simulink model "Bringup"  (R2024b)
settings: Solver=FixedStepDiscrete  StartTime=0.0  StopTime=Inf  FixedStep=Ts0  RelTol=1e-3  EnableMultiTasking=on
undefined symbols (not defined in the file): Omega, Ts0, Ts0Single
libraries: svdschedulerlib x1
settings Model: DataDictionary=RectData.sldd  VariantConfigurationObject=Conf  ExtModeTrigDuration=8  Creator=sgade  LastModifiedBy=sgade
settings SolverCC: AutoInsertRateTranBlk=on
settings OptimizationCC: DefaultUnderspecifiedDataType=single  EnhancedBackFolding=on  PassReuseOutputArgsAs=Individual arguments  MaxStackSize=1024  OptimizeBlockOrder=speed  DifferentSizesBufferReuse=on  OptimizationCustomize=off  EfficientTunableParamExpr=on
settings DebuggingCC: ParameterTunabilityLossMsg=error
settings HardwareCC: ProdBitPerChar=16  ProdBitPerInt=16  ProdBitPerPointer=32  ProdBitPerSizeT=32  ProdBitPerPtrDiffT=32  ProdLargestAtomicInteger=Integer  ProdLargestAtomicFloat=None  ProdWordSize=16  ProdLongLongMode=on  ProdHWDeviceType=Texas Instruments->C2000
settings SFSimCC: MATLABDynamicMemAlloc=off
settings RTWCC: Description=Embedded Coder  SystemTargetFile=ert.tlc  HardwareBoard=TI F280013x  TemplateMakefile=ert_default_tmf  Toolchain=Texas Instruments Code Composer Studio (C2000)  CodeProfilingSaveOptions=MetricsOnly
settings CodeAppCC: ForceParamTrailComments=on  IgnoreCustomStorageClasses=off  OperatorAnnotations=on  SimulinkDataObjDesc=on  SFDataObjDesc=on  InsertBlockDesc=on
settings ERTTargetCC: CodeReplacementLibrary=TI C28x  ExtModeTransport=4  ExtModeStaticAlloc=on  ExtModeAutomaticAllocSize=off  ExtModeStaticAllocSize=1000  ExtModeMexFile=ext_xcp  ExtModeIntrfLevel=Level2 - Open  InlinedParameterPlacement=Hierarchical  EnableUserReplacementTypes=on

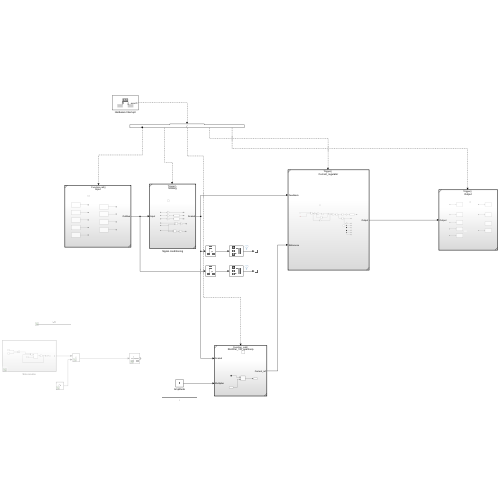
[thumbnail: Simulink's stored preview of the top-level diagram]
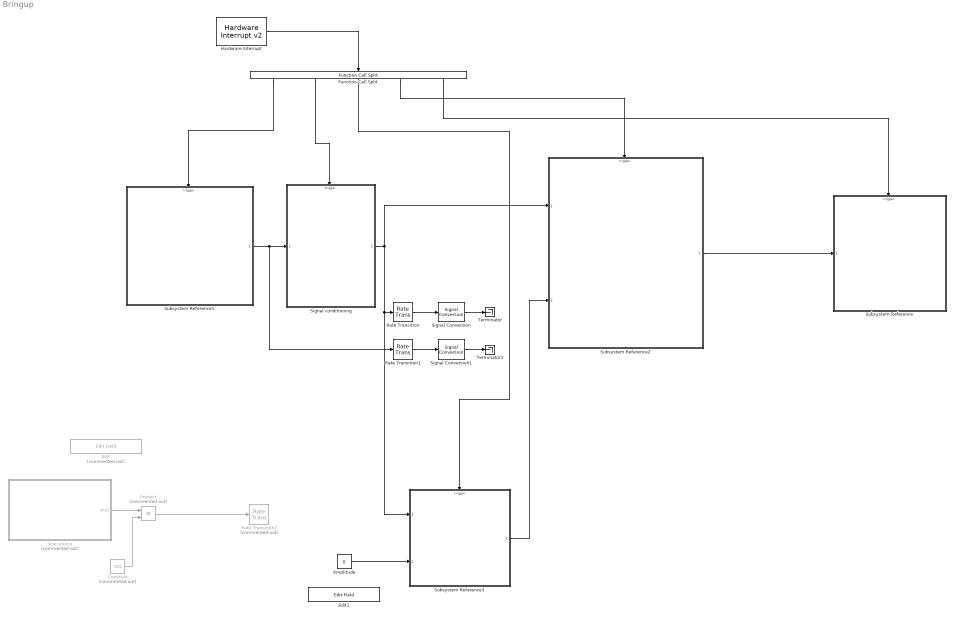
== system Bringup ==
  Amplitude : Constant  Value=0  OutDataTypeStr=single
  Constant : Constant  Commented=on  Value=125
  Edit : EditField  Commented=on  LabelPosition=Hide  ShowInitialText=on  Alignment=Center
  Edit1 : EditField  LabelPosition=Hide  ShowInitialText=on  Alignment=Center
  Function-Call Split : FunctionCallSplit  IconShape=distinctive  NumOutputPorts=5  OutputPortLayout=default
  Hardware Interrupt : svdschedulerlib/Hardware Interrupt v2  ISRGroup=ADC - Analog to Digital Converter  ISRName=ADCA1_INT  ISRNumber=32  NumEventsToServe=1  EventsList={'on','EOC event','1';'off','Overflow event','2';'off','Custom event','3'}  SelectedEvents={'event1'}  TaskPriority=50  DisablePreemption=off  ClearInterruptFlagsAtEndOfEvent=on  InterruptDefinitionFile=$(TARGET_ROOT)/registry/interrupts/F2837xS_interrupts.xml  HardwareBoard=F2837x  EnableSimPort=off
      settings: LibrarySourceBlock=c2000lib/Scheduling/Hardware Interrupt
  Product : Product  Commented=on
  Rate Transition : RateTransition  Deterministic=off  OutPortSampleTime=1/1000
  Rate Transition1 : RateTransition  Deterministic=off  OutPortSampleTime=1/1000
  Rate Transition2 : RateTransition  Commented=on  Deterministic=off
  Signal Conversion : SignalConversion  OverrideOpt=off
  Signal Conversion1 : SignalConversion  OverrideOpt=off
  Signal conditioning : Subsystem  ReferencedSubsystem=Scaling
      settings: PermitHierarchicalResolution=None
  Sine source : Subsystem  Commented=on
  Subsystem Reference : Subsystem  ReferencedSubsystem=Output
      settings: PermitHierarchicalResolution=None
  Subsystem Reference1 : Subsystem  ReferencedSubsystem=Input
  Subsystem Reference2 : Subsystem  ReferencedSubsystem=Current_regulator
      settings: PermitHierarchicalResolution=None
  Subsystem Reference3 : Subsystem  ReferencedSubsystem=Rectifier_VR_openloop
      settings: PermitHierarchicalResolution=None
  Terminator : Terminator
  Terminator1 : Terminator
  wires:
  Signal Conversion/1 -> Terminator/1
  Subsystem Reference2/1 -> Subsystem Reference/1
  Rate Transition/1 -> Signal Conversion/1
  Function-Call Split/1 -> Subsystem Reference1/Trigger
  Function-Call Split/2 -> Signal conditioning/Trigger
  Signal conditioning/1 -> Subsystem Reference2/1, Subsystem Reference3/1, Rate Transition/1
  Hardware Interrupt/1 -> Function-Call Split/1
  Subsystem Reference1/1 -> Rate Transition1/1, Signal conditioning/1
  Signal Conversion1/1 -> Terminator1/1
  Rate Transition1/1 -> Signal Conversion1/1
  Sine source/1(Out1) -> Product/1
  Constant/1 -> Product/2
  Product/1 -> Rate Transition2/1
  Function-Call Split/5 -> Subsystem Reference/Trigger
  Function-Call Split/4 -> Subsystem Reference2/Trigger
  Function-Call Split/3 -> Subsystem Reference3/Trigger
  Subsystem Reference3/1 -> Subsystem Reference2/2
  Amplitude/1 -> Subsystem Reference3/2

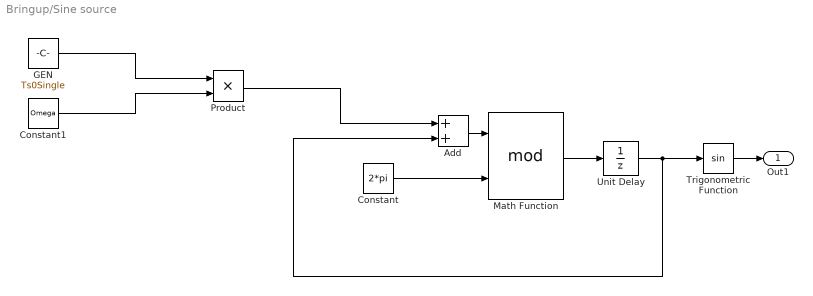
== system Bringup/Sine source ==
  Add : Sum
  Constant : Constant  Value=2*pi  OutDataTypeStr=single
  Constant1 : Constant  Value=Omega  SampleTime=Ts0
  GEN : Constant  Value=Ts0Single  OutDataTypeStr=single  SampleTime=Ts0
  Math Function : Math  Operator=mod
  Product : Product
  Trigonometric Function : Trigonometry
  Unit Delay : UnitDelay  SampleTime=-1  HasFrameUpgradeWarning=on
  Out1 : Outport
  wires:
  GEN/1 -> Product/1
  Unit Delay/1 -> Trigonometric Function/1, Add/2
  Product/1 -> Add/1
  Constant/1 -> Math Function/2
  Trigonometric Function/1 -> Out1/1
  Math Function/1 -> Unit Delay/1
  Constant1/1 -> Product/2
  Add/1 -> Math Function/1
